simulink model "greenhouse_discrete"  (R2018a)
settings: Solver=VariableStepAuto  StartTime=0.0  StopTime=24*60*60  RelTol=1e-3
values from neighbouring files (symbols this model uses):
  A = 1    [init.m]
  a_B = 3.3e-6    (= 3.3e-06)    [init.m]
  a_C = 1000    [init.m]
  a_H = 1    [init.m]
  a_T = 1/12000    (= 8.33333333333e-05)    [init.m]
  a_W = 5    [init.m]
  alpha = 2e-5    (= 2e-05)    [init.m]
  b_B = 5.0e-6    (= 5e-06)    [init.m]
  b_C = 17    [init.m]
  b_H = 2    [init.m]
  b_T = 1/600    (= 0.00166666666667)    [init.m]
  b_W = 8.3e-6    (= 8.3e-06)    [init.m]
  beta = 2.3e-5    (= 2.3e-05)    [init.m]
  c_B = 7.0e-9    (= 7e-09)    [init.m]
  c_C = 2.8e-8    (= 2.8e-08)    [init.m]
  c_H = 3e-4    (= 0.0003)    [init.m]
  C_init = 930    [init.m]
  C_ReferencePoint = 900    [init.m]
  c_T = 1/12000    (= 8.33333333333e-05)    [init.m]
  c_W = 1    [init.m]
  d_B = 1.8e-7    (= 1.8e-07)    [init.m]
  d_C = 5.6e-2    (= 0.056)    [init.m]
  d_H = 12    [init.m]
  d_W = 1    [init.m]
  gamma = 0.002    [init.m]
  H_init = 70    [init.m]
  H_ReferencePoint = 75    [init.m]
  nu = 1.4e-5    (= 1.4e-05)    [init.m]
  T_init = 20    [init.m]
  T_opt = 22    [init.m]
  W_init = 65    [init.m]
  W_ReferencePoint = 70    [init.m]
libraries: simulink x3
settings Model: Creator=Mahsa  LastModifiedBy=Mahsa

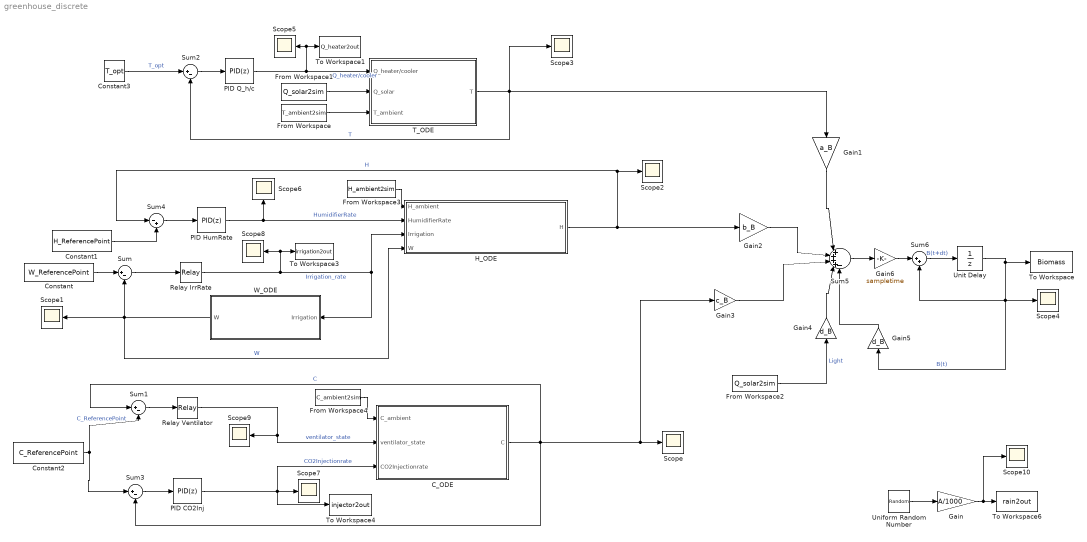
== system greenhouse_discrete ==
  C_ODE : Subsystem
  Constant : Constant  Value=W_ReferencePoint  SampleTime=sampletime
  Constant1 : Constant  Value=H_ReferencePoint  SampleTime=sampletime
  Constant2 : Constant  Value=C_ReferencePoint  SampleTime=sampletime
  Constant3 : Constant  Value=T_opt  SampleTime=sampletime
  From Workspace : FromWorkspace  VariableName=T_ambient2sim  SampleTime=sampletime
  From Workspace1 : FromWorkspace  VariableName=Q_solar2sim  SampleTime=sampletime
  From Workspace2 : FromWorkspace  VariableName=Q_solar2sim  SampleTime=sampletime
  From Workspace3 : FromWorkspace  VariableName=H_ambient2sim  SampleTime=sampletime
  From Workspace4 : FromWorkspace  VariableName=C_ambient2sim  SampleTime=sampletime
  Gain : Gain  Gain=A/1000
  Gain1 : Gain  Gain=a_B
  Gain2 : Gain  Gain=b_B
  Gain3 : Gain  Gain=c_B
  Gain4 : Gain  Gain=d_B
  Gain5 : Gain  Gain=d_B
  Gain6 : Gain  Gain=sampletime
  "H_ODE " : Subsystem
  PID CO2Inj : simulink/Continuous/PID Controller  Controller=PID  TimeDomain=Discrete-time  SampleTime=sampletime  IntegratorMethod=Forward Euler  FilterMethod=Forward Euler  Form=Parallel  UseFilter=on  ControllerParametersSource=internal  P=4.93391858283706e-05  I=3.20108230742453e-06  D=-2.73242197427014e-05  N=0.124965561480679  InitialConditionSource=internal  InitialConditionForIntegrator=0  InitialConditionForFilter=0  ExternalReset=none  LimitOutput=on  UpperSaturationLimit=inf  LowerSaturationLimit=0  LinearizeAsGain=on  AntiWindupMode=none  Kb=1  TrackingMode=off  Kt=1  PParamMin=[]  PParamMax=[]  IParamMin=[]  IParamMax=[]  DParamMin=[]  DParamMax=[]  NParamMin=[]  NParamMax=[]  KbParamMin=[]  KbParamMax=[]  KtParamMin=[]  KtParamMax=[]  POutMin=[]  POutMax=[]  IOutMin=[]  IOutMax=[]  DOutMin=[]  DOutMax=[]  NOutMin=[]  NOutMax=[]  KbOutMin=[]  KbOutMax=[]  KtOutMin=[]  KtOutMax=[]  IntegratorOutMin=[]  IntegratorOutMax=[]  FilterOutMin=[]  FilterOutMax=[]  SumOutMin=[]  SumOutMax=[]  SumI1OutMin=[]  SumI1OutMax=[]  SumI2OutMin=[]  SumI2OutMax=[]  SumI3OutMin=[]  SumI3OutMax=[]  SumDOutMin=[]  SumDOutMax=[]  SaturationOutMin=[]  SaturationOutMax=[]  IntegratorContinuousStateAttributes=''  IntegratorStateMustResolveToSignalObject=off  IntegratorRTWStateStorageClass=Auto  FilterContinuousStateAttributes=''  FilterStateMustResolveToSignalObject=off  FilterRTWStateStorageClass=Auto  DifferentiatorICPrevScaledInput=0  DifferentiatorOutMin=[]  DifferentiatorOutMax=[]  FilterDiffOutCoefMin=[]  FilterDiffOutCoefMax=[]  SumDenOutMin=[]  SumDenOutMax=[]  SumNumOutMin=[]  SumNumOutMax=[]  ReciprocalOutMin=[]  ReciprocalOutMax=[]  DivideOutMin=[]  DivideOutMax=[]  TunerSelectOption=Transfer Function Based (PID Tuner App)
  PID HumRate : simulink/Continuous/PID Controller  Controller=PID  TimeDomain=Discrete-time  SampleTime=sampletime  IntegratorMethod=Forward Euler  FilterMethod=Forward Euler  Form=Parallel  UseFilter=on  ControllerParametersSource=internal  P=3.39270173476506e-05  I=2.04480190627856e-08  D=-0.00379979861644551  N=0.00114765941857276  InitialConditionSource=internal  InitialConditionForIntegrator=0  InitialConditionForFilter=0  ExternalReset=none  LimitOutput=off  UpperSaturationLimit=inf  LowerSaturationLimit=-inf  LinearizeAsGain=on  AntiWindupMode=none  Kb=1  TrackingMode=off  Kt=1  PParamMin=[]  PParamMax=[]  IParamMin=[]  IParamMax=[]  DParamMin=[]  DParamMax=[]  NParamMin=[]  NParamMax=[]  KbParamMin=[]  KbParamMax=[]  KtParamMin=[]  KtParamMax=[]  POutMin=[]  POutMax=[]  IOutMin=[]  IOutMax=[]  DOutMin=[]  DOutMax=[]  NOutMin=[]  NOutMax=[]  KbOutMin=[]  KbOutMax=[]  KtOutMin=[]  KtOutMax=[]  IntegratorOutMin=[]  IntegratorOutMax=[]  FilterOutMin=[]  FilterOutMax=[]  SumOutMin=[]  SumOutMax=[]  SumI1OutMin=[]  SumI1OutMax=[]  SumI2OutMin=[]  SumI2OutMax=[]  SumI3OutMin=[]  SumI3OutMax=[]  SumDOutMin=[]  SumDOutMax=[]  SaturationOutMin=[]  SaturationOutMax=[]  IntegratorContinuousStateAttributes=''  IntegratorStateMustResolveToSignalObject=off  IntegratorRTWStateStorageClass=Auto  FilterContinuousStateAttributes=''  FilterStateMustResolveToSignalObject=off  FilterRTWStateStorageClass=Auto  DifferentiatorICPrevScaledInput=0  DifferentiatorOutMin=[]  DifferentiatorOutMax=[]  FilterDiffOutCoefMin=[]  FilterDiffOutCoefMax=[]  SumDenOutMin=[]  SumDenOutMax=[]  SumNumOutMin=[]  SumNumOutMax=[]  ReciprocalOutMin=[]  ReciprocalOutMax=[]  DivideOutMin=[]  DivideOutMax=[]  TunerSelectOption=Transfer Function Based (PID Tuner App)
  PID Q_h/c : simulink/Continuous/PID Controller  Controller=PID  TimeDomain=Discrete-time  SampleTime=sampletime  IntegratorMethod=Forward Euler  FilterMethod=Forward Euler  Form=Parallel  UseFilter=on  ControllerParametersSource=internal  P=26.6328130643636  I=0.0891686910196959  D=-511.482477785438  N=0.00506771888250834  InitialConditionSource=internal  InitialConditionForIntegrator=0  InitialConditionForFilter=0  ExternalReset=none  LimitOutput=off  UpperSaturationLimit=inf  LowerSaturationLimit=-inf  LinearizeAsGain=on  AntiWindupMode=none  Kb=1  TrackingMode=off  Kt=1  PParamMin=[]  PParamMax=[]  IParamMin=[]  IParamMax=[]  DParamMin=[]  DParamMax=[]  NParamMin=[]  NParamMax=[]  KbParamMin=[]  KbParamMax=[]  KtParamMin=[]  KtParamMax=[]  POutMin=[]  POutMax=[]  IOutMin=[]  IOutMax=[]  DOutMin=[]  DOutMax=[]  NOutMin=[]  NOutMax=[]  KbOutMin=[]  KbOutMax=[]  KtOutMin=[]  KtOutMax=[]  IntegratorOutMin=[]  IntegratorOutMax=[]  FilterOutMin=[]  FilterOutMax=[]  SumOutMin=[]  SumOutMax=[]  SumI1OutMin=[]  SumI1OutMax=[]  SumI2OutMin=[]  SumI2OutMax=[]  SumI3OutMin=[]  SumI3OutMax=[]  SumDOutMin=[]  SumDOutMax=[]  SaturationOutMin=[]  SaturationOutMax=[]  IntegratorContinuousStateAttributes=''  IntegratorStateMustResolveToSignalObject=off  IntegratorRTWStateStorageClass=Auto  FilterContinuousStateAttributes=''  FilterStateMustResolveToSignalObject=off  FilterRTWStateStorageClass=Auto  DifferentiatorICPrevScaledInput=0  DifferentiatorOutMin=[]  DifferentiatorOutMax=[]  FilterDiffOutCoefMin=[]  FilterDiffOutCoefMax=[]  SumDenOutMin=[]  SumDenOutMax=[]  SumNumOutMin=[]  SumNumOutMax=[]  ReciprocalOutMin=[]  ReciprocalOutMax=[]  DivideOutMin=[]  DivideOutMax=[]  TunerSelectOption=Transfer Function Based (PID Tuner App)
  Relay IrrRate : Relay  OnSwitchValue=10  OffSwitchValue=-10  OnOutputValue=IrrigationRate
  Relay Ventilator : Relay  OnSwitchValue=100  OffSwitchValue=-100
  Scope{,1..10} (11 alike) : Scope
  Sum{,1..3} (4 alike) : Sum  Inputs=|+-
  Sum4 : Sum  Inputs=|-+
  Sum5 : Sum  Inputs=|++++-
  Sum6 : Sum  Inputs=|++
  T_ODE : Subsystem
  To Workspace : ToWorkspace  VariableName=Biomass  SaveFormat=Timeseries  SampleTime=sampletime
  To Workspace1 : ToWorkspace  VariableName=Q_heater2out  SaveFormat=Timeseries  SampleTime=sampletime
  To Workspace3 : ToWorkspace  VariableName=irrigation2out  SaveFormat=Timeseries  SampleTime=sampletime
  To Workspace4 : ToWorkspace  VariableName=injector2out  SaveFormat=Timeseries  SampleTime=sampletime
  To Workspace6 : ToWorkspace  VariableName=rain2out  SaveFormat=Timeseries  SampleTime=sampletime
  Uniform Random Number : UniformRandomNumber  Minimum=0  Maximum=0.01  SampleTime=3600
  Unit Delay : UnitDelay  SampleTime=sampletime
  "W_ODE " : Subsystem
  wires:
  Sum2/1 -> PID Q_h/c/1
  Constant3/1 -> Sum2/1  "T_opt"
  T_ODE/1("T ") -> Scope3/1, Sum2/2, Gain1/1  "T"
  PID Q_h/c/1 -> T_ODE/1(Q_heater/cooler), To Workspace1/1, Scope5/1  "Q_heater/cooler"
  Unit Delay/1 -> Gain5/1, Scope4/1, Sum6/2, To Workspace/1  "B(t)"
  Sum5/1 -> Gain6/1
  Sum/1 -> Relay IrrRate/1
  Constant/1 -> Sum/1
  "W_ODE "/1("W ") -> "H_ODE "/4(W), Scope1/1, Sum/2  "W"
  Relay IrrRate/1 -> Scope8/1, To Workspace3/1, "H_ODE "/3("Irrigation "), "W_ODE "/1(Irrigation)  "Irrigation_rate"
  PID HumRate/1 -> "H_ODE "/2(HumidifierRate), Scope6/1  "HumidifierRate"
  "H_ODE "/1("H ") -> Gain2/1, Scope2/1, Sum4/1  "H"
  Constant1/1 -> Sum4/2
  Sum4/1 -> PID HumRate/1
  Constant2/1 -> Sum3/1, Sum1/2  "C_ReferencePoint"
  Sum1/1 -> Relay Ventilator/1
  Sum3/1 -> PID CO2Inj/1
  Relay Ventilator/1 -> C_ODE/2(ventilator_state), Scope9/1  "ventilator_state"
  PID CO2Inj/1 -> Scope7/1, C_ODE/3(CO2Injectionrate), To Workspace4/1  "CO2Injectionrate"
  C_ODE/1(C) -> Scope/1, Gain3/1, Sum1/1, Sum3/2  "C"
  Gain1/1 -> Sum5/1
  Gain2/1 -> Sum5/2
  Gain3/1 -> Sum5/3
  From Workspace2/1 -> Gain4/1  "Light"
  Gain4/1 -> Sum5/4
  Gain5/1 -> Sum5/5
  From Workspace1/1 -> T_ODE/2(Q_solar)
  From Workspace/1 -> T_ODE/3(T_ambient)
  From Workspace3/1 -> "H_ODE "/1(H_ambient)
  From Workspace4/1 -> C_ODE/1(C_ambient)
  Uniform Random Number/1 -> Gain/1
  Gain/1 -> Scope10/1, To Workspace6/1
  Gain6/1 -> Sum6/1
  Sum6/1 -> Unit Delay/1  "B(t+dt)"

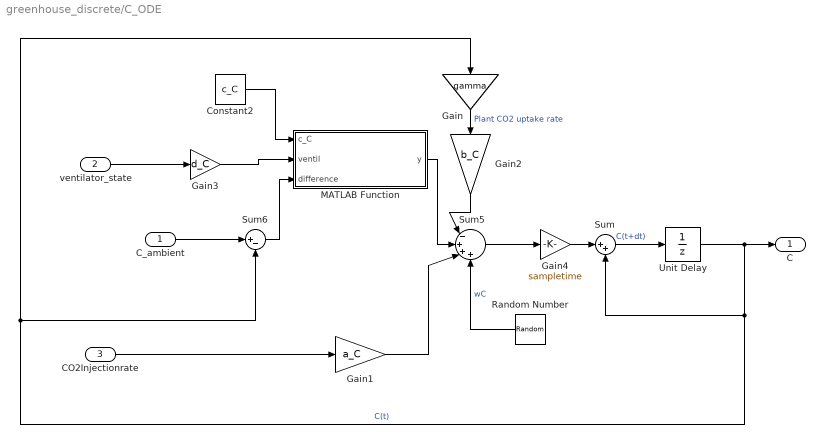
== system greenhouse_discrete/C_ODE ==
  C_ambient : Inport
  ventilator_state : Inport  Port=2
  CO2Injectionrate : Inport  Port=3
  Constant2 : Constant  Value=c_C
  Gain : Gain  Gain=gamma
  Gain1 : Gain  Gain=a_C
  Gain2 : Gain  Gain=b_C
  Gain3 : Gain  Gain=d_C
  Gain4 : Gain  Gain=sampletime
  MATLAB Function : MATLAB Function  TreatAsAtomicUnit=on
  Random Number : RandomNumber  SampleTime=sampletime
  Sum : Sum  Inputs=|++
  Sum5 : Sum  Inputs=|-+++
  Sum6 : Sum  Inputs=|+-
  Unit Delay : UnitDelay  InitialCondition=C_init  SampleTime=sampletime
  C : Outport
  wires:
  Gain2/1 -> Sum5/1
  MATLAB Function/1(y) -> Sum5/2
  Random Number/1 -> Sum5/4  "wC"
  Gain3/1 -> MATLAB Function/2(ventil)
  Sum5/1 -> Gain4/1
  C_ambient/1 -> Sum6/1
  Gain1/1 -> Sum5/3
  Constant2/1 -> MATLAB Function/1(c_C)
  Gain/1 -> Gain2/1  "Plant CO2 uptake rate"
  CO2Injectionrate/1 -> Gain1/1
  Unit Delay/1 -> Sum/2, Gain/1, Sum6/2, C/1  "C(t)"
  ventilator_state/1 -> Gain3/1
  Sum6/1 -> MATLAB Function/3(difference)
  Gain4/1 -> Sum/1
  Sum/1 -> Unit Delay/1  "C(t+dt)"

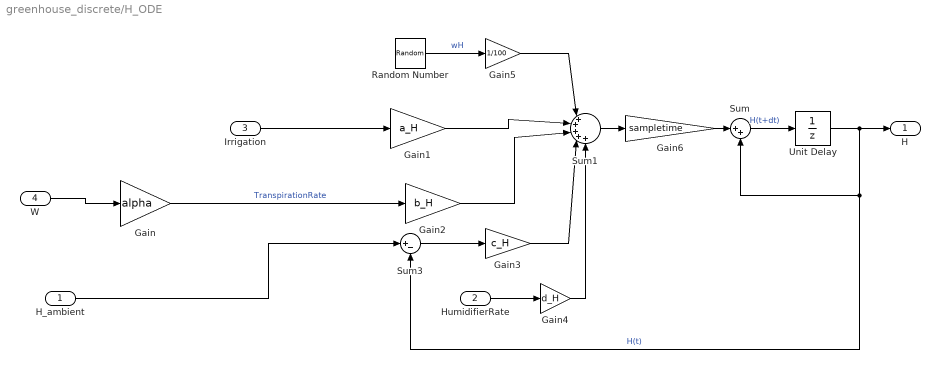
== system greenhouse_discrete/H_ODE  ==
  H_ambient : Inport
  HumidifierRate : Inport  Port=2
  "Irrigation " : Inport  Port=3
  W : Inport  Port=4
  Gain : Gain  Gain=alpha
  Gain1 : Gain  Gain=a_H
  Gain2 : Gain  Gain=b_H
  Gain3 : Gain  Gain=c_H
  Gain4 : Gain  Gain=d_H
  Gain5 : Gain  Gain=1/100
  Gain6 : Gain  Gain=sampletime
  Random Number : RandomNumber  SampleTime=sampletime
  Sum : Sum  Inputs=|++
  Sum1 : Sum  Inputs=|+++++
  Sum3 : Sum  Inputs=|+-
  Unit Delay : UnitDelay  InitialCondition=H_init  SampleTime=sampletime
  "H " : Outport
  wires:
  Sum3/1 -> Gain3/1
  Gain2/1 -> Sum1/3
  "Irrigation "/1 -> Gain1/1
  Gain1/1 -> Sum1/2
  Gain3/1 -> Sum1/4
  HumidifierRate/1 -> Gain4/1
  Sum1/1 -> Gain6/1
  Gain4/1 -> Sum1/5
  H_ambient/1 -> Sum3/1
  Gain/1 -> Gain2/1  "TranspirationRate"
  Unit Delay/1 -> Sum/2, Sum3/2, "H "/1  "H(t)"
  W/1 -> Gain/1
  Random Number/1 -> Gain5/1  "wH"
  Gain5/1 -> Sum1/1
  Gain6/1 -> Sum/1
  Sum/1 -> Unit Delay/1  "H(t+dt)"

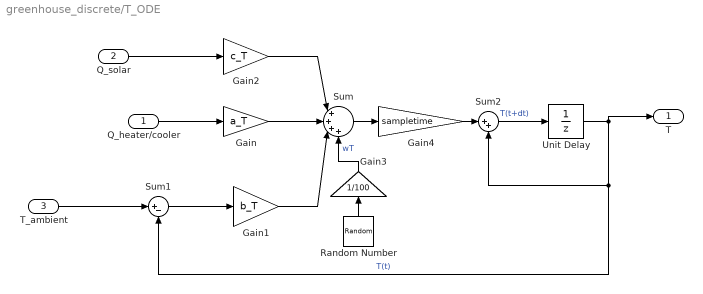
== system greenhouse_discrete/T_ODE ==
  Q_heater/cooler : Inport
  Q_solar : Inport  Port=2
  T_ambient : Inport  Port=3
  Gain : Gain  Gain=a_T
  Gain1 : Gain  Gain=b_T
  Gain2 : Gain  Gain=c_T
  Gain3 : Gain  Gain=1/100
  Gain4 : Gain  Gain=sampletime
  Random Number : RandomNumber  SampleTime=sampletime
  Sum : Sum  Inputs=|++++
  Sum1 : Sum  Inputs=|+-
  Sum2 : Sum  Inputs=|++
  Unit Delay : UnitDelay  InitialCondition=T_init  SampleTime=sampletime
  "T " : Outport
  wires:
  Q_solar/1 -> Gain2/1
  Q_heater/cooler/1 -> Gain/1
  Sum1/1 -> Gain1/1
  Gain1/1 -> Sum/3
  Gain2/1 -> Sum/1
  Gain/1 -> Sum/2
  T_ambient/1 -> Sum1/1
  Unit Delay/1 -> "T "/1, Sum2/2, Sum1/2  "T(t)"
  Gain3/1 -> Sum/4  "wT"
  Random Number/1 -> Gain3/1
  Sum/1 -> Gain4/1
  Gain4/1 -> Sum2/1
  Sum2/1 -> Unit Delay/1  "T(t+dt)"

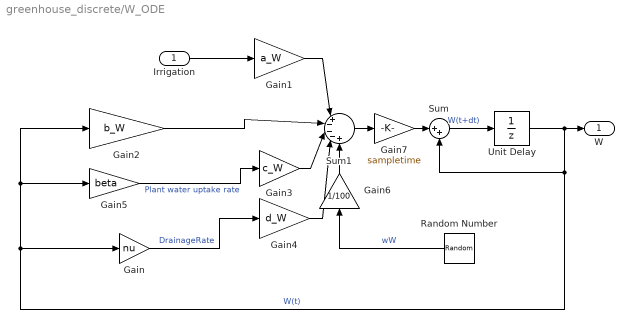
== system greenhouse_discrete/W_ODE  ==
  Irrigation : Inport
  Gain : Gain  Gain=nu
  Gain1 : Gain  Gain=a_W
  Gain2 : Gain  Gain=b_W
  Gain3 : Gain  Gain=c_W
  Gain4 : Gain  Gain=d_W
  Gain5 : Gain  Gain=beta
  Gain6 : Gain  Gain=1/100
  Gain7 : Gain  Gain=sampletime
  Random Number : RandomNumber  SampleTime=sampletime
  Sum : Sum  Inputs=|++
  Sum1 : Sum  Inputs=|+---+
  Unit Delay : UnitDelay  InitialCondition=W_init  SampleTime=sampletime
  "W " : Outport
  wires:
  Gain/1 -> Gain4/1  "DrainageRate"
  Gain3/1 -> Sum1/3
  Gain5/1 -> Gain3/1  "Plant water uptake rate"
  Gain2/1 -> Sum1/2
  Gain1/1 -> Sum1/1
  Gain4/1 -> Sum1/4
  Irrigation/1 -> Gain1/1
  Unit Delay/1 -> Sum/2, Gain2/1, Gain5/1, Gain/1, "W "/1  "W(t)"
  Random Number/1 -> Gain6/1  "wW"
  Gain6/1 -> Sum1/5
  Sum1/1 -> Gain7/1
  Gain7/1 -> Sum/1
  Sum/1 -> Unit Delay/1  "W(t+dt)"

== matlab function greenhouse_discrete/C_ODE/MATLAB Function ==
  data: c_C input; y output; ventil input; difference input
function y = fcn(c_C, ventil, difference)

y = (c_C+ventil).*difference;
